simulink model "FuzzyPIDControl"  (R2016b)
settings: Solver=VariableStepAuto  StartTime=0.0  StopTime=60  RelTol=1e-3
undefined symbols (not defined in the file): myFis
libraries: fuzblock x1
settings Model: Creator=xuzong  LastModifiedBy=xuzong
settings SolverCC: MaxConsecutiveMinStep=0.1  ZeroCrossControl=DisableAll  ZeroCrossAlgorithm=Adaptive

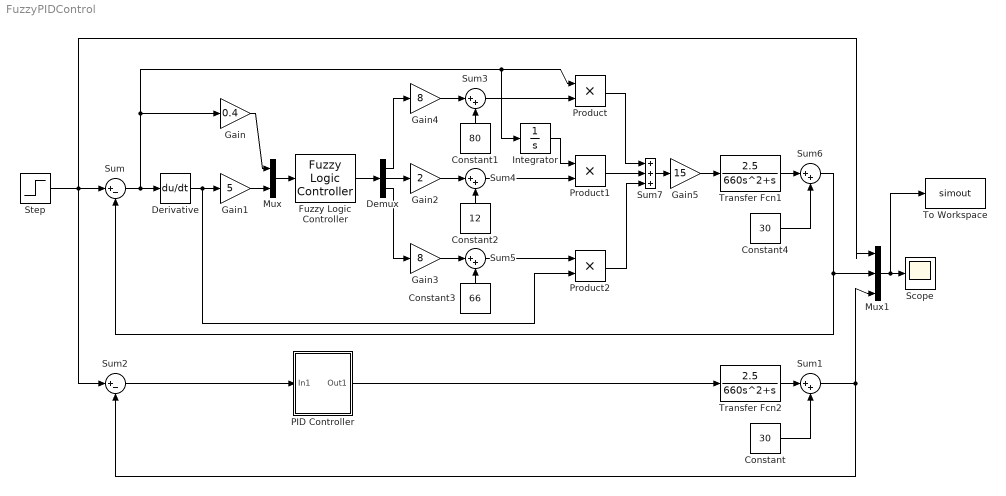
== system FuzzyPIDControl ==
  Constant : Constant  Value=30
  Constant1 : Constant  Value=80
  Constant2 : Constant  Value=12
  Constant3 : Constant  Value=66
  Constant4 : Constant  Value=30
  Demux : Demux  Outputs=3
  Derivative : Derivative
  Fuzzy Logic Controller : fuzblock/Fuzzy Logic  Controller  fis=[myFis]
  Gain : Gain  Gain=0.4
  Gain1 : Gain  Gain=5
  Gain2 : Gain  Gain=2
  Gain3 : Gain  Gain=8
  Gain4 : Gain  Gain=8
  Gain5 : Gain  Gain=15
  Integrator : Integrator
  Mux : Mux  Inputs=2
  Mux1 : Mux  Inputs=3
  PID Controller : Subsystem
      mask Display: disp('PID\nController')
  Product : Product
  Product1 : Product
  Product2 : Product
  Scope : Scope
  Step : Step  Time=0  Before=30  After=50  SampleTime=0
  Sum : Sum  Inputs=|+-
  Sum{1,3..6} (5 alike) : Sum  Inputs=|++
  Sum2 : Sum  Inputs=|+-
  Sum7 : Sum  Inputs=+++
  To Workspace : ToWorkspace  VariableName=simout  SaveFormat=Timeseries  SampleTime=-1
      settings: Decimation=3
  Transfer Fcn1 : TransferFcn  Numerator=[2.5]  Denominator=[660 1 0]
  Transfer Fcn2 : TransferFcn  Numerator=[2.5]  Denominator=[660 1 0]
  wires:
  Sum2/1 -> PID Controller/1(In1)
  Transfer Fcn2/1 -> Sum1/1
  Constant/1 -> Sum1/2
  Sum1/1 -> Mux1/3, Sum2/2
  Mux1/1 -> To Workspace/1, Scope/1
  Step/1 -> Sum/1, Mux1/1, Sum2/1
  Gain1/1 -> Mux/2
  Gain/1 -> Mux/1
  Mux/1 -> Fuzzy Logic Controller/1
  Fuzzy Logic Controller/1 -> Demux/1
  Demux/2 -> Gain2/1
  Demux/1 -> Gain4/1
  Demux/3 -> Gain3/1
  Gain4/1 -> Sum3/1
  Gain2/1 -> Sum4/1
  Gain3/1 -> Sum5/1
  Constant1/1 -> Sum3/2
  Constant2/1 -> Sum4/2
  Constant3/1 -> Sum5/2
  Sum3/1 -> Product/2
  Sum/1 -> Product/1, Integrator/1, Gain/1, Derivative/1
  Integrator/1 -> Product1/1
  Sum4/1 -> Product1/2
  Sum5/1 -> Product2/1
  Derivative/1 -> Product2/2, Gain1/1
  Product1/1 -> Sum7/2
  Product/1 -> Sum7/1
  Product2/1 -> Sum7/3
  Gain5/1 -> Transfer Fcn1/1
  Constant4/1 -> Sum6/2
  Transfer Fcn1/1 -> Sum6/1
  Sum6/1 -> Mux1/2, Sum/2
  Sum7/1 -> Gain5/1
  PID Controller/1(Out1) -> Transfer Fcn2/1

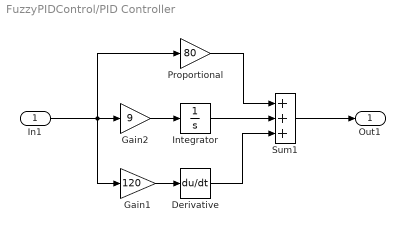
== system FuzzyPIDControl/PID Controller ==
  In1 : Inport
  Derivative : Derivative
  Gain1 : Gain  Gain=120
  Gain2 : Gain  Gain=9
  Integrator : Integrator
  Proportional : Gain  Gain=80
  Sum1 : Sum  Inputs=+++
  Out1 : Outport
  wires:
  In1/1 -> Proportional/1, Gain1/1, Gain2/1
  Proportional/1 -> Sum1/1
  Gain1/1 -> Derivative/1
  Sum1/1 -> Out1/1
  Integrator/1 -> Sum1/2
  Derivative/1 -> Sum1/3
  Gain2/1 -> Integrator/1
